simulink model "iddempr5"  (Simulink 4.00)
settings: Solver=ode45  StartTime=0.0  StopTime=500  RelTol=1e-3
libraries: simulink3 x1
settings Model: LimitDataPoints=off  IntegerOverflowMsg=none  ExtModeTrigMode=oneshot  ExtModeArmWhenConnect=off

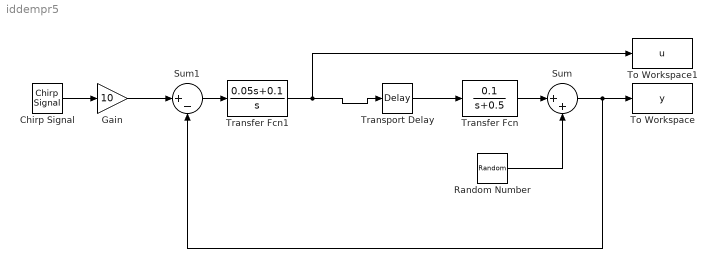
== system iddempr5 ==
  Chirp Signal : simulink3/Sources/Chirp Signal  f1=0.001  T=500  f2=0.2
  Gain : Gain  Gain=10  Multiplication=Element-wise(K.*u)  SaturateOnIntegerOverflow=on
  Random Number : RandomNumber  Mean=0  Variance=0.01  Seed=0  SampleTime=0.5
  Sum : Sum  Inputs=|++  SaturateOnIntegerOverflow=on
  Sum1 : Sum  Inputs=|+-  SaturateOnIntegerOverflow=on
  To Workspace : ToWorkspace  VariableName=y  SampleTime=0.5  SaveFormat=Array
  To Workspace1 : ToWorkspace  VariableName=u  SampleTime=0.5  SaveFormat=Array
  Transfer Fcn : TransferFcn  Numerator=0.1  Denominator=[1 0.5]  AbsoluteTolerance=auto  Realization=auto
  Transfer Fcn1 : TransferFcn  Numerator=[0.05 0.1]  Denominator=[1 0]  AbsoluteTolerance=auto  Realization=auto
  Transport Delay : TransportDelay  DelayTime=1.57  InitialInput=0  BufferSize=1024  PadeOrder=0
  wires:
  Transport Delay/1 -> Transfer Fcn/1
  Transfer Fcn/1 -> Sum/1
  Random Number/1 -> Sum/2
  Sum1/1 -> Transfer Fcn1/1
  Sum/1 -> To Workspace/1, Sum1/2
  Chirp Signal/1 -> Gain/1
  Gain/1 -> Sum1/1
  Transfer Fcn1/1 -> Transport Delay/1, To Workspace1/1
